simulink model "pvinverter_det_pmref"  (R2014a)
settings: Solver=FixedStepDiscrete  StartTime=0.0  StopTime=0.2  FixedStep=Ts  MaxStep=1e-3  RelTol=1e-4
PreLoadFcn:
  | PVArrayIsc = 5;
  | PVArrayVoc = 21.6;
  | PVArrayRs = 0.036;
  | Tcircuit = 27.15;
  | Toffset = -2;
  | TIPH1 = 0.001;
  | TXIS1 = 3;
  | TRS1 = 0;
  | Ts = 1e-6;
  | load('InvBusObject');
  | load('PVBusObject');
InitFcn:
  | Ts = 1e-6;
StartFcn:
  | tic;
StopFcn:
  | toc;
undefined symbols (not defined in the file or in its folder): sigbuilder_block
settings Model: Creator=cosorio  LastModifiedBy=cosorio
settings DataIOCC: LimitDataPoints=off  SignalLoggingSaveFormat=ModelDataLogs  SaveOutput=off  SignalLogging=off  SaveTime=off
settings OptimizationCC: InlineParams=on  ExpressionDepthLimit=2147483647
settings DebuggingCC: UnderspecifiedInitializationDetection=Classic  SolverPrmCheckMsg=none  FcnCallInpInsideContextMsg=UseLocalSettings  StateNameClashWarn=warning
settings GRTTargetCC: CombineOutputUpdateFcns=off  GRTInterface=on

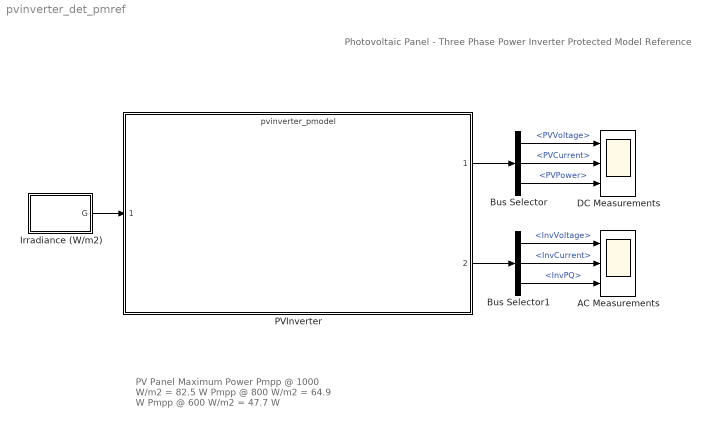
== system pvinverter_det_pmref ==
  note: Photovoltaic Panel - Three Phase Power Inverter
      | Protected Model Reference
  note: PV Panel Maximum Power
      | Pmpp @ 1000 W/m2 = 82.5 W
      | Pmpp @ 800 W/m2 = 64.9 W
      | Pmpp @ 600 W/m2 = 47.7 W
  AC Measurements : Scope  NumInputPorts=3
      settings: YMin=-10~-10~0  YMax=10~10~100  SaveName=InverterData
  Bus Selector : BusSelector  OutputSignals=PVVoltage,PVCurrent,PVPower
  Bus Selector1 : BusSelector  OutputSignals=InvVoltage,InvCurrent,InvPQ
  DC Measurements : Scope  NumInputPorts=3
      settings: YMin=0~0~0  YMax=25~6~100
  Irradiance (W/m2) : Subsystem  Tag=STV Subsys  LoadFcn=sigbuilder_block('load');  StartFcn=sigbuilder_block('start');  StopFcn=sigbuilder_block('stop');  ClipboardFcn=sigbuilder_block('clipboard');  mask(Sigbuilder block){}
      mask help: Sigbuilder GUI
      mask init:
      | if ~strcmp(get_param(bdroot(gcbh),'SimulationStatus'),'stopped') tuvar = sigbuilder_block('maskInit'); end
      settings: CopyFcn=sigbuilder_block('copy');  DeleteFcn=sigbuilder_block('delete');  ModelCloseFcn=sigbuilder_block('modelClose');  PreSaveFcn=sigbuilder_block('preSave');  PauseFcn=sigbuilder_block('pause')  ContinueFcn=sigbuilder_block('continue')  NameChangeFcn=sigbuilder_block('namechange');  OpenFcn=sigbuilder_block('open',[124.138 46.5517 550.552 391.034 ]);  CloseFcn=sigbuilder_block('close');
      mask Display: plot(0,0,100,100,[10,10,40,40,10],[80,20,20,80,80],[40,10],[50,50], [40,27,10],[65,72,56],[40,25,25,10],[28,28,43,43]);
  PVInverter : ModelReference  ModelNameDialog=pvinverter_pmodel.slxp  ModelReferenceVersion=1.198  CopyOfModelName=pvinverter_pmodel.slxp  CopyOfModelProtected=on  DefaultDataLogging=off
  wires:
  Bus Selector/3 -> DC Measurements/3  "<PVPower>"
  Bus Selector/1 -> DC Measurements/1  "<PVVoltage>"
  Bus Selector/2 -> DC Measurements/2  "<PVCurrent>"
  Bus Selector1/1 -> AC Measurements/1  "<InvVoltage>"
  Bus Selector1/2 -> AC Measurements/2  "<InvCurrent>"
  Bus Selector1/3 -> AC Measurements/3  "<InvPQ>"
  Irradiance (W/m2)/1(G) -> PVInverter/1
  PVInverter/1 -> Bus Selector/1
  PVInverter/2 -> Bus Selector1/1

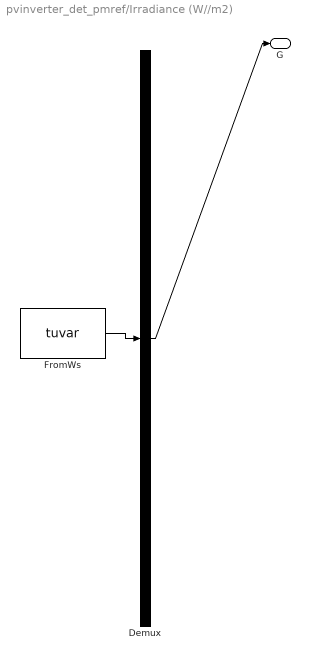
== system pvinverter_det_pmref/Irradiance (W//m2) ==
  Demux : Demux  Tag=STV Demux  Outputs=1
  FromWs : FromWorkspace  Tag=STV FromWs  VariableName=tuvar  SampleTime=Ts
      SigBuilderData=|
      | common.afterFinalStr = 'Extrapolate'
      | common.sampleTime = 'Ts'
      | dataSet(1).timeRange = [0 1]
      | dataSet(1).name = 'Constant Irradiance'
      | dataSet(2).timeRange = [0 1]
      | dataSet(2).name = 'Step Irradiance'
      | dataSet(3).timeRange = [0 1]
      | dataSet(3).name = 'Trapezoidal Irradiance'
      | sbobj.Groups(1).Name = 'Constant Irradiance'
      | sbobj.Groups(1).Signals.Name = 'G'
      | sbobj.Groups(1).Signals.XData = [0 1]
      | sbobj.Groups(1).Signals.YData = [800 800]
      | sbobj.Groups(1).TimeRange = [0 1]
      | sbobj.Groups(2).Name = 'Step Irradiance'
      | sbobj.Groups(2).Signals.Name = 'G'
      | sbobj.Groups(2).Signals.XData = [0 0.5 0.5 1]
      | sbobj.Groups(2).Signals.YData = [600 600 1000 1000]
      | sbobj.Groups(2).TimeRange = [0 1]
      | sbobj.Groups(3).Name = 'Trapezoidal Irradiance'
      | sbobj.Groups(3).Signals.Name = 'G'
      | sbobj.Groups(3).Signals.XData = [0 0.2 0.3 0.5 0.7 0.9 1]
      | sbobj.Groups(3).Signals.YData = [800 800 600 600 1000 1000 800]
      | sbobj.Groups(3).TimeRange = [0 1]
  G : Outport  Tag=STV Outport
  wires:
  Demux/1 -> G/1
  FromWs/1 -> Demux/1
